simulink model "exp4"  (R2025b)
settings: Solver=VariableStepAuto  StartTime=0.0  StopTime=10.0  RelTol=1e-3
settings Model: Creator=SUBHASH  LastModifiedBy=SUBHASH

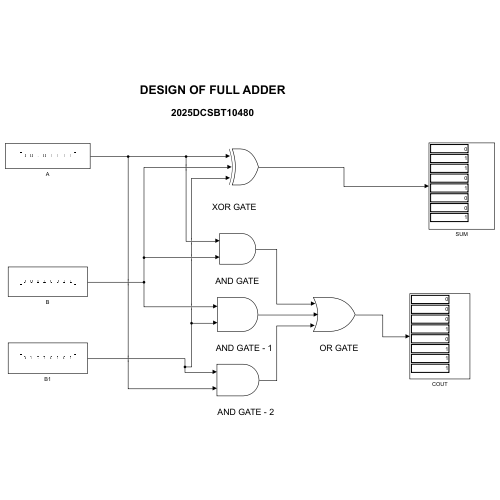
[thumbnail: Simulink's stored preview of the top-level diagram]
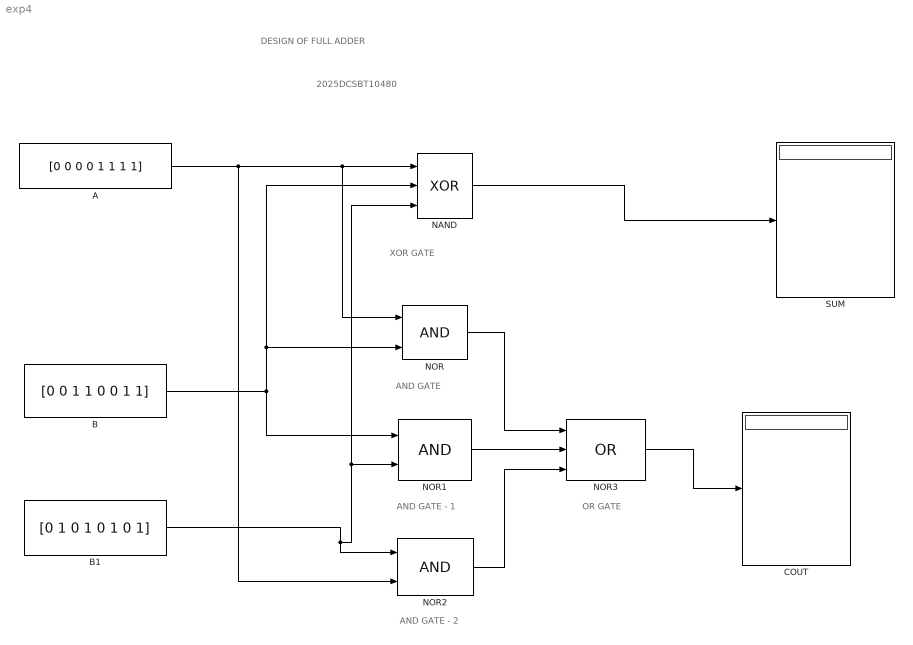
== system exp4 ==
  note: 2025DCSBT10480
  note: DESIGN OF FULL ADDER
  note: AND GATE
  note: XOR GATE
  note: OR GATE
  note: AND GATE - 1
  note: AND GATE - 2
  A : Constant  Value=[0 0 0 0 1 1 1 1]
  B : Constant  Value=[0 0 1 1 0 0 1 1]
  B1 : Constant  Value=[0 1 0 1 0 1 0 1]
  COUT : Display
      settings: Decimation=8
  NAND : Logic  Operator=XOR  Inputs=3  IconShape=distinctive  AllPortsSameDT=off  OutDataTypeStr=boolean
  NOR : Logic  IconShape=distinctive  AllPortsSameDT=off  OutDataTypeStr=boolean
  NOR1 : Logic  IconShape=distinctive  AllPortsSameDT=off  OutDataTypeStr=boolean
  NOR2 : Logic  IconShape=distinctive  AllPortsSameDT=off  OutDataTypeStr=boolean
  NOR3 : Logic  Operator=OR  Inputs=3  IconShape=distinctive  AllPortsSameDT=off  OutDataTypeStr=boolean
  SUM : Display
      settings: Decimation=8
  wires:
  B/1 -> NOR1/1, NAND/2, NOR/2
  NAND/1 -> SUM/1
  B1/1 -> NOR2/1, NOR1/2, NAND/3
  A/1 -> NOR2/2, NOR/1, NAND/1
  NOR/1 -> NOR3/1
  NOR1/1 -> NOR3/2
  NOR2/1 -> NOR3/3
  NOR3/1 -> COUT/1
